simulink model "ROCR6II_URDF_file_915"  (R2020b)
settings: Solver=VariableStepAuto  StartTime=0.0  StopTime=10  FixedStep=0.01  RelTol=1e-3
values from neighbouring files (symbols this model uses):
  X = [x,y,z,Roll,Pitch,Yaw]    [T2RPY.m]
undefined symbols (not defined in the file or in its folder): A, Y, Z
libraries: fl_lib x115, sm_lib x74, nesl_utility x59, fl_ps_legacy_lib x48, ee_lib x12, simulink_extras x7, simulink x6
(part 1 of 5)
settings Model: Creator=Jeason  LastModifiedBy=GDXYY-006-F
settings DataIOCC: ReturnWorkspaceOutputs=off
settings DebuggingCC: ArithmeticOperatorsInVariantConditions=warning
settings SFSimCC: CustomCodeUndefinedFunction=UseInterfaceOnly

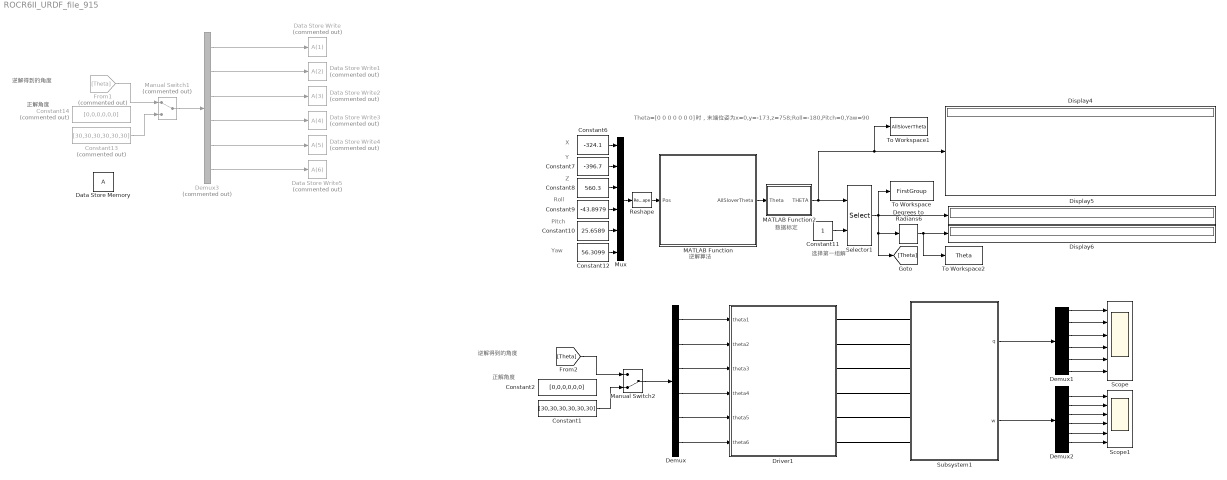
== system ROCR6II_URDF_file_915 ==
  note: 选择第一组解
  note: 数据标定
  note: Theta=[0 0 0 0 0 0 0]时，末端位姿为x=0,y=-173,z=758;Roll=-180,Pitch=0,Yaw=90
  note: 逆解算法
  note: 正解角度
  note: 逆解得到的角度
  note: Y
  note: Yaw
  note: Pitch
  note: Roll
  note: X
  note: Z
  note: 正解角度
  note: 逆解得到的角度
  Constant1 : Constant  Value=[30,30,30,30,30,30]
  Constant10 : Constant  Value=25.6589
  Constant11 : Constant
  Constant12 : Constant  Value=56.3099
  Constant13 : Constant  Commented=on  Value=[30,30,30,30,30,30]
  Constant14 : Constant  Commented=on  Value=[0,0,0,0,0,0]
  Constant2 : Constant  Value=[0,0,0,0,0,0]
  Constant6 : Constant  Value=-324.1
  Constant7 : Constant  Value=-396.7
  Constant8 : Constant  Value=560.3
  Constant9 : Constant  Value=-43.8979
  Data Store Write : DataStoreWrite  Commented=on  DataStoreElements=A(1)
  Data Store Write1 : DataStoreWrite  Commented=on  DataStoreElements=A(2)
  Data Store Write2 : DataStoreWrite  Commented=on  DataStoreElements=A(3)
  Data Store Write3 : DataStoreWrite  Commented=on  DataStoreElements=A(4)
  Data Store Write4 : DataStoreWrite  Commented=on  DataStoreElements=A(5)
  Data Store Write5 : DataStoreWrite  Commented=on  DataStoreElements=A(6)
  Data Store Memory : DataStoreMemory  ReadBeforeWriteMsg=warning  WriteAfterWriteMsg=warning  WriteAfterReadMsg=warning  InitialValue=[0 0 0 0 0 0]  ShowAdditionalParam=off
  Degrees to Radians6 : simulink_extras/Transformations/Degrees to Radians
  Demux : Demux  Outputs=6
  Demux1 : Demux  Outputs=6
  Demux2 : Demux  Outputs=6
  Demux3 : Demux  Commented=on  Outputs=6
  Display4 : Display
  Display5 : Display
  Display6 : Display
  Driver1 : Subsystem  mask{angle1=0, angle2=0, angle3=0, angle4=0, angle5=0, angle6=0}
      mask prompts: angle1 "InitTheta1(deg)"; angle2 "InitTheta2(deg)"; angle3 "InitTheta3(deg)"; angle4 "InitTheta4(deg)"; angle5 "InitTheta5(deg)"; angle6 "InitTheta6(deg)"
  From1 : From  Commented=on  GotoTag=Theta
  MATLAB Function : MATLAB Function  TreatAsAtomicUnit=on
  MATLAB Function2 : MATLAB Function  TreatAsAtomicUnit=on
  Manual Switch1 : ManualSwitch  Commented=on
  Manual Switch2 : ManualSwitch  CurrentSetting=0
  Mux : Mux  Inputs=6
  Reshape : Reshape  OutputDimensionality=Customize  OutputDimensions=[1,6]
  Scope : Scope  NumInputPorts=6
  Scope1 : Scope  NumInputPorts=6
  Selector1 : Selector  NumberOfDimensions=2  InputPortWidth=10  IndexOptions=Index vector (port),Starting index (dialog)  Indices=[1 3],1  OutputSizes=1,6
  Subsystem1 : Subsystem
  To Workspace : ToWorkspace  VariableName=FirstGroup  SampleTime=-1
      settings: MaxDataPoints=1
  To Workspace1 : ToWorkspace  VariableName=AllSloverTheta  SampleTime=-1
      settings: MaxDataPoints=1
  To Workspace2 : ToWorkspace  VariableName=Theta  SampleTime=-1
      settings: MaxDataPoints=1
  wires:
  Demux2/4 -> Scope1/4
  Demux1/4 -> Scope/4
  Demux2/6 -> Scope1/6
  Demux1/1 -> Scope/1
  Demux2/5 -> Scope1/5
  Demux2/1 -> Scope1/1
  Subsystem1/2(w) -> Demux2/1
  Demux2/3 -> Scope1/3
  Demux1/6 -> Scope/6
  Demux2/2 -> Scope1/2
  Demux1/2 -> Scope/2
  Subsystem1/1(q) -> Demux1/1
  Demux1/3 -> Scope/3
  Demux1/5 -> Scope/5
  Demux/1 -> Driver1/1(theta1)
  Demux/2 -> Driver1/2(theta2)
  Demux/3 -> Driver1/3(theta3)
  Demux/4 -> Driver1/4(theta4)
  Demux/5 -> Driver1/5(theta5)
  Demux/6 -> Driver1/6(theta6)
  Selector1/1 -> Display5/1, Degrees to Radians6/1, [Theta], To Workspace/1
  Degrees to Radians6/1 -> Display6/1, To Workspace2/1
  Reshape/1 -> MATLAB Function/1(Pos)
  Constant11/1 -> Selector1/2
  Mux/1 -> Reshape/1
  MATLAB Function/1(AllSloverTheta) -> MATLAB Function2/1(Theta)
  MATLAB Function2/1(THETA) -> Selector1/1, Display4/1, To Workspace1/1
  Constant13/1 -> Manual Switch1/2
  From1/1 -> Manual Switch1/1
  Demux3/4 -> Data Store Write3/1
  Demux3/6 -> Data Store Write5/1
  Demux3/1 -> Data Store Write/1
  Demux3/2 -> Data Store Write1/1
  Demux3/3 -> Data Store Write2/1
  Manual Switch1/1 -> Demux3/1
  Demux3/5 -> Data Store Write4/1
  Constant8/1 -> Mux/3
  Constant10/1 -> Mux/5
  Constant7/1 -> Mux/2
  Constant12/1 -> Mux/6
  Constant6/1 -> Mux/1
  Constant9/1 -> Mux/4
  Manual Switch2/1 -> Demux/1
  [Theta] -> Manual Switch2/1
  Constant1/1 -> Manual Switch2/2
  connections:
  Driver1/RConn1 -- Subsystem1/LConn1
  Driver1/RConn2 -- Subsystem1/LConn2
  Driver1/RConn3 -- Subsystem1/LConn3
  Driver1/RConn4 -- Subsystem1/LConn4
  Driver1/RConn5 -- Subsystem1/LConn5
  Driver1/RConn6 -- Subsystem1/LConn6

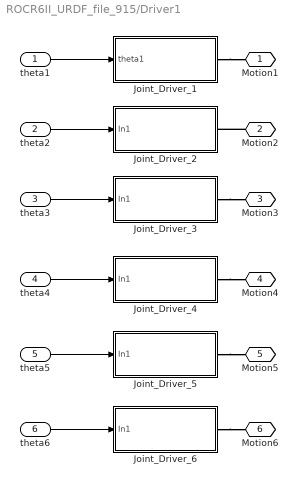
== system ROCR6II_URDF_file_915/Driver1 ==
  theta1 : Inport
  theta2 : Inport  Port=2
  theta3 : Inport  Port=3
  theta4 : Inport  Port=4
  theta5 : Inport  Port=5
  theta6 : Inport  Port=6
  Joint_Driver_1 : Subsystem
  Joint_Driver_2 : Subsystem
  Joint_Driver_3 : Subsystem
  Joint_Driver_4 : Subsystem
  Joint_Driver_5 : Subsystem
  Joint_Driver_6 : Subsystem
  Motion1 : PMIOPort  Side=Right
  Motion2 : PMIOPort  Port=2  Side=Right
  Motion3 : PMIOPort  Port=3  Side=Right
  Motion4 : PMIOPort  Port=4  Side=Right
  Motion5 : PMIOPort  Port=5  Side=Right
  Motion6 : PMIOPort  Port=6  Side=Right
  wires:
  theta2/1 -> Joint_Driver_2/1(In1)
  theta3/1 -> Joint_Driver_3/1(In1)
  theta4/1 -> Joint_Driver_4/1(In1)
  theta6/1 -> Joint_Driver_6/1(In1)
  theta5/1 -> Joint_Driver_5/1(In1)
  theta1/1 -> Joint_Driver_1/1(theta1)
  connections:
  Motion2/RConn1 -- Joint_Driver_2/RConn1
  Joint_Driver_6/RConn1 -- Motion6/RConn1
  Joint_Driver_1/RConn1 -- Motion1/RConn1
  Joint_Driver_3/RConn1 -- Motion3/RConn1
  Joint_Driver_5/RConn1 -- Motion5/RConn1
  Joint_Driver_4/RConn1 -- Motion4/RConn1

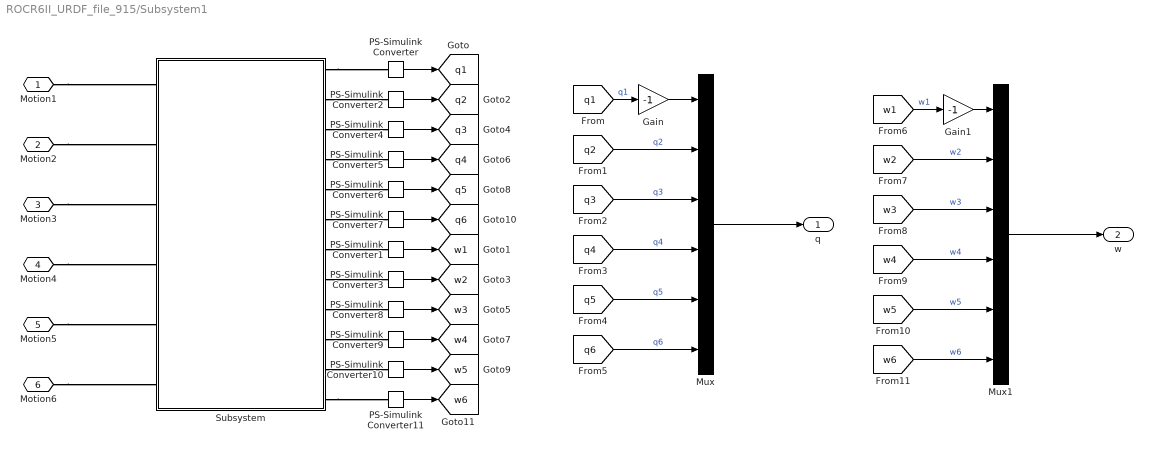
== system ROCR6II_URDF_file_915/Subsystem1 ==
  Gain : Gain  Gain=-1
  Gain1 : Gain  Gain=-1
  Mux : Mux  Inputs=6
  Mux1 : Mux  Inputs=6
  PS-Simulink Converter{,2,4..7} (6 alike) : nesl_utility/PS-Simulink Converter  PhysicalDomain=network_engine_domain  SubClassName=ps_output  LeftPortType=input  RightPortType=output  PseudoPeriodic=off  Frequencies=[]  Unit=deg  AffineConversion=off
  PS-Simulink Converter{1,3,8..11} (6 alike) : nesl_utility/PS-Simulink Converter  PhysicalDomain=network_engine_domain  SubClassName=ps_output  LeftPortType=input  RightPortType=output  PseudoPeriodic=off  Frequencies=[]  Unit=deg/s  AffineConversion=off
  Subsystem : Subsystem
  Motion1 : PMIOPort  Side=Left
  Motion2 : PMIOPort  Port=2  Side=Left
  Motion3 : PMIOPort  Port=3  Side=Left
  Motion4 : PMIOPort  Port=4  Side=Left
  Motion5 : PMIOPort  Port=5  Side=Left
  Motion6 : PMIOPort  Port=6  Side=Left
  q : Outport
  w : Outport  Port=2
  tag scope: q1=global, q2=global, q3=global, q4=global, q5=global, q6=global, w1=global, w2=global, w3=global, w4=global, w5=global, w6=global
  wires:
  [q2] -> Mux/2  "q2"
  PS-Simulink Converter11/1 -> [w6]
  PS-Simulink Converter1/1 -> [w1]
  Mux/1 -> q/1
  [w1] -> Gain1/1  "w1"
  PS-Simulink Converter6/1 -> [q5]
  [w4] -> Mux1/4  "w4"
  PS-Simulink Converter/1 -> [q1]
  [q6] -> Mux/6  "q6"
  PS-Simulink Converter7/1 -> [q6]
  [q3] -> Mux/3  "q3"
  [q4] -> Mux/4  "q4"
  PS-Simulink Converter10/1 -> [w5]
  PS-Simulink Converter4/1 -> [q3]
  PS-Simulink Converter2/1 -> [q2]
  [w2] -> Mux1/2  "w2"
  PS-Simulink Converter9/1 -> [w4]
  PS-Simulink Converter8/1 -> [w3]
  PS-Simulink Converter3/1 -> [w2]
  [w6] -> Mux1/6  "w6"
  Mux1/1 -> w/1
  [w5] -> Mux1/5  "w5"
  Gain1/1 -> Mux1/1
  PS-Simulink Converter5/1 -> [q4]
  Gain/1 -> Mux/1
  [w3] -> Mux1/3  "w3"
  [q1] -> Gain/1  "q1"
  [q5] -> Mux/5  "q5"
  connections:
  Subsystem/RConn12 -- PS-Simulink Converter11/LConn1
  Subsystem/RConn8 -- PS-Simulink Converter3/LConn1
  Subsystem/RConn4 -- PS-Simulink Converter5/LConn1
  Subsystem/RConn1 -- PS-Simulink Converter/LConn1
  Subsystem/RConn11 -- PS-Simulink Converter10/LConn1
  Subsystem/RConn2 -- PS-Simulink Converter2/LConn1
  Subsystem/RConn5 -- PS-Simulink Converter6/LConn1
  Subsystem/RConn3 -- PS-Simulink Converter4/LConn1
  Subsystem/RConn9 -- PS-Simulink Converter8/LConn1
  Subsystem/RConn7 -- PS-Simulink Converter1/LConn1
  Subsystem/RConn10 -- PS-Simulink Converter9/LConn1
  Subsystem/RConn6 -- PS-Simulink Converter7/LConn1
  Motion1/RConn1 -- Subsystem/LConn1
  Motion2/RConn1 -- Subsystem/LConn2
  Motion3/RConn1 -- Subsystem/LConn3
  Motion4/RConn1 -- Subsystem/LConn4
  Motion5/RConn1 -- Subsystem/LConn5
  Motion6/RConn1 -- Subsystem/LConn6

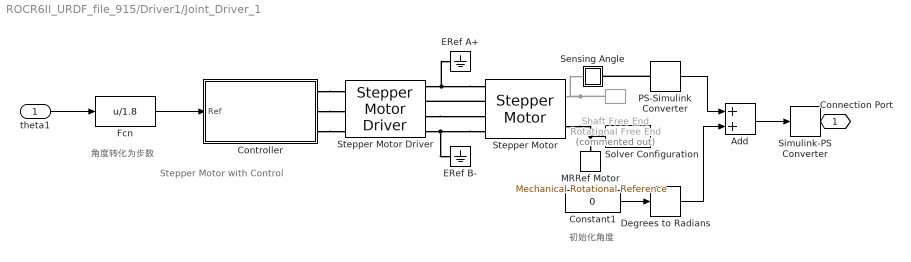
== system ROCR6II_URDF_file_915/Driver1/Joint_Driver_1 ==
  note: 初始化角度
  note: Stepper Motor with Control
  note: 角度转化为步数
  theta1 : Inport
  Add : Sum
  Constant1 : Constant  Value=0
  Controller : Subsystem  Variant=on  VariantControlMode=label  LabelModeActiveChoice=Position
      settings: AttributesFormatString=%<BlockChoice>
  Degrees to Radians : simulink_extras/Transformations/Degrees to Radians
  ERef A+ : fl_lib/Electrical/Electrical Elements/Electrical Reference
      settings: SourceProductName=Foundation Library
  ERef B- : fl_lib/Electrical/Electrical Elements/Electrical Reference
      settings: SourceProductName=Foundation Library
  Fcn : Fcn  Expr=u/1.8
  MRRef Motor : fl_lib/Mechanical/Rotational Elements/Mechanical Rotational Reference
      settings: SourceProductName=Foundation Library
  PS-Simulink Converter : nesl_utility/PS-Simulink Converter  PhysicalDomain=network_engine_domain  SubClassName=ps_output  LeftPortType=input  RightPortType=output  PseudoPeriodic=off  Frequencies=[]  Unit=1  AffineConversion=off
  Sensing Angle : Subsystem
      mask Display: disp('a')
  Shaft Free End : fl_lib/Mechanical/Rotational Elements/Rotational Free End  Commented=on  w_specify=off  w_priority=None  w=0 rad/s  w_nominal_specify=off  w_nominal_unit=rad/s  w_nominal_value=1
      settings: SourceProductName=Foundation Library
  Simulink-PS Converter : nesl_utility/Simulink-PS Converter  PhysicalDomain=network_engine_domain  SubClassName=ps_input  LeftPortType=input  RightPortType=output  PseudoPeriodic=off  Frequencies=[]  NoiseDistribution=none  NoiseParameters=[]  Unit=1  AffineConversion=off  FilteringAndDerivatives=filter  SimscapeFilterOrder=2  InputFilterTimeConstant=0.001  UdotUserProvided=0
  Solver Configuration : nesl_utility/Solver Configuration  PhysicalDomain=network_engine_domain  SubClassName=solver  LeftPortType=input  RightPortType=generic  Tones=[]  Harmonics=[]  SimulateNoise=off  Profile=off  UseLocalSampling=off  EnableSwitchedLinearOptims=on  FrequencyDomain=off  UseCCode=off  RelTol=0.001  AbsTol=1e-06  MinStep=1e-09  ToWorkspace=off  RevertToSquareIcSolve=off  NumHomotopyIterations=100  PhasorMode=off  PhasorModeNumHarmonics=1  DoDC=off  ResidualTolerance=1e-9  UseLocalSolver=off  LocalSolverChoice=NE_BACKWARD_EULER_ADVANCER  LocalSolverSampleTime=.001  DoFixedCost=off  MaxNonlinIter=3  MaxModeIter=2  ComputeImpulses=off  ImpulseIterations=2  LinearAlgebra=Sparse  EquationFormulation=NE_TIME_EF  DelaysMemoryBudget=1024  AutomaticFiltering=on  FilteringTimeConstant=0.001  PartitionStorageMethod=AS_NEEDED  PartitionMemoryBudget=1024  PartitionMethod=FAST
  Stepper Motor : ee_lib/Electromechanical/Reluctance & Stepper/Stepper Motor  step_or_av=1  w_vec=[ 0 1000 3e+3 ] rpm  T_vec=[ 2 2 1 ] N*m  assert_if_slipping=0  J_total=1e-4 kg*m^2  max_step_rate=10 Hz  Ra=0.55 Ohm  La=0.0015 H  Km=0.19 N*m/A  Td=0 N*m  Rm=Inf Ohm  Step=1.8 deg  J=4.5e-05 kg*m^2  B=1e-02 N*m/(rad/s)  speed0=0 rpm  theta0=0 deg  alpha=[.00393, .00393] 1/K  Tmeas=25 degC  T_vec2=[1.7, 1.7, .85] N*m  Tmeas2=125 degC  half_stepping=0  thermal_masses=[100, 100] J/K  initial_temperatures=[25, 25] degC  rotor_thermal_mass=50 J/K  rotor_initial_temperature=25 degC  Rm_percent_rotor=90
      settings: SourceProductBaseCode=PS  InternalSimscapePortConfiguration="{\"Bottom\":[],\"Left\":[{\"id\":\"pA\",\"label\":\"A+\",\"type\":\"foundation.electrical.electrical\"},{\"id\":\"nA\",\"label\":\"A-\",\"type\":\"foundation.electrical.electrical\"},{\"id\":\"pB\",\"label\":\"B+\",\"type\":\"foundation.electrical.electrical\"},{\"id\":\"nB\",\"label\":\"B-\",\"type\":\"foundation.electrical.electrical\"}],\"Right\":[{\"id\":\"R\",\"label\":\"R\",\"type\":\"foundation.mechanical.rotational.rotational\"},{\"id\":\"C\",\"label\":\"C\",\"type\":\"foundation.mechanical.rotational.rotational\"}],\"Top\":[]}"
  Stepper Motor Driver : ee_lib/Electromechanical/Reluctance & Stepper/Stepper Motor Driver  step_or_av=1  step_rate_per_volt=10 Hz/V  Venable=2.5 V  Vreverse=2.5 V  Vm=5 V  half_stepping=0
      settings: SourceProductBaseCode=PS  InternalSimscapePortConfiguration="{\"Bottom\":[],\"Left\":[{\"id\":\"ENA\",\"label\":\"ENA\",\"type\":\"foundation.electrical.electrical\"},{\"id\":\"REF\",\"label\":\"REF\",\"type\":\"foundation.electrical.electrical\"},{\"id\":\"REV\",\"label\":\"REV\",\"type\":\"foundation.electrical.electrical\"}],\"Right\":[{\"id\":\"pA\",\"label\":\"A+\",\"type\":\"foundation.electrical.electrical\"},{\"id\":\"nA\",\"label\":\"A-\",\"type\":\"foundation.electrical.electrical\"},{\"id\":\"pB\",\"label\":\"B+\",\"type\":\"foundation.electrical.electrical\"},{\"id\":\"nB\",\"label\":\"B-\",\"type\":\"foundation.electrical.electrical\"}],\"Top\":[]}"
  Connection Port : PMIOPort  Side=Right
  wires:
  Fcn/1 -> Controller/1(Ref)
  theta1/1 -> Fcn/1
  Constant1/1 -> Degrees to Radians/1
  PS-Simulink Converter/1 -> Add/1
  Add/1 -> Simulink-PS Converter/1
  Degrees to Radians/1 -> Add/2
  connections:
  PS-Simulink Converter/LConn1 -- Sensing Angle/RConn1
  Controller/RConn3 -- Stepper Motor Driver/LConn3
  Controller/RConn2 -- Stepper Motor Driver/LConn2
  Controller/RConn1 -- Stepper Motor Driver/LConn1
  Stepper Motor/LConn2 -- Stepper Motor Driver/RConn2
  Stepper Motor Driver/RConn3 -- Stepper Motor/LConn3
  Stepper Motor/LConn1 -- Stepper Motor Driver/RConn1 -- ERef A+/LConn1
  Solver Configuration/RConn1 -- Stepper Motor/RConn2 -- MRRef Motor/LConn1
  Shaft Free End/LConn1 -- Sensing Angle/LConn1 -- Stepper Motor/RConn1
  Stepper Motor/LConn4 -- Stepper Motor Driver/RConn4 -- ERef B-/LConn1
  Connection Port/RConn1 -- Simulink-PS Converter/RConn1

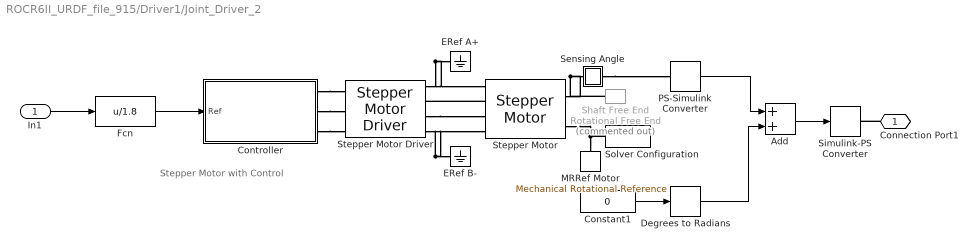
== system ROCR6II_URDF_file_915/Driver1/Joint_Driver_2 ==
  note: Stepper Motor with Control
  In1 : Inport
  Add : Sum
  Constant1 : Constant  Value=0
  Controller : Subsystem  Variant=on  VariantControlMode=label  LabelModeActiveChoice=Position
      settings: AttributesFormatString=%<BlockChoice>
  Degrees to Radians : simulink_extras/Transformations/Degrees to Radians
  ERef A+ : fl_lib/Electrical/Electrical Elements/Electrical Reference
      settings: SourceProductName=Foundation Library
  ERef B- : fl_lib/Electrical/Electrical Elements/Electrical Reference
      settings: SourceProductName=Foundation Library
  Fcn : Fcn  Expr=u/1.8
  MRRef Motor : fl_lib/Mechanical/Rotational Elements/Mechanical Rotational Reference
      settings: SourceProductName=Foundation Library
  PS-Simulink Converter : nesl_utility/PS-Simulink Converter  PhysicalDomain=network_engine_domain  SubClassName=ps_output  LeftPortType=input  RightPortType=output  PseudoPeriodic=off  Frequencies=[]  Unit=1  AffineConversion=off
  Sensing Angle : Subsystem
      mask Display: disp('a')
  Shaft Free End : fl_lib/Mechanical/Rotational Elements/Rotational Free End  Commented=on  w_specify=off  w_priority=None  w=0 rad/s  w_nominal_specify=off  w_nominal_unit=rad/s  w_nominal_value=1
      settings: SourceProductName=Foundation Library
  Simulink-PS Converter : nesl_utility/Simulink-PS Converter  PhysicalDomain=network_engine_domain  SubClassName=ps_input  LeftPortType=input  RightPortType=output  PseudoPeriodic=off  Frequencies=[]  NoiseDistribution=none  NoiseParameters=[]  Unit=1  AffineConversion=off  FilteringAndDerivatives=filter  SimscapeFilterOrder=2  InputFilterTimeConstant=0.001  UdotUserProvided=0
  Solver Configuration : nesl_utility/Solver Configuration  PhysicalDomain=network_engine_domain  SubClassName=solver  LeftPortType=input  RightPortType=generic  Tones=[]  Harmonics=[]  SimulateNoise=off  Profile=off  UseLocalSampling=off  EnableSwitchedLinearOptims=on  FrequencyDomain=off  UseCCode=off  RelTol=0.001  AbsTol=1e-06  MinStep=1e-09  ToWorkspace=off  RevertToSquareIcSolve=off  NumHomotopyIterations=100  PhasorMode=off  PhasorModeNumHarmonics=1  DoDC=off  ResidualTolerance=1e-9  UseLocalSolver=off  LocalSolverChoice=NE_BACKWARD_EULER_ADVANCER  LocalSolverSampleTime=.001  DoFixedCost=off  MaxNonlinIter=3  MaxModeIter=2  ComputeImpulses=off  ImpulseIterations=2  LinearAlgebra=Sparse  EquationFormulation=NE_TIME_EF  DelaysMemoryBudget=1024  AutomaticFiltering=on  FilteringTimeConstant=0.001  PartitionStorageMethod=AS_NEEDED  PartitionMemoryBudget=1024  PartitionMethod=FAST
  Stepper Motor : ee_lib/Electromechanical/Reluctance & Stepper/Stepper Motor  step_or_av=1  w_vec=[ 0 1000 3e+3 ] rpm  T_vec=[ 2 2 1 ] N*m  assert_if_slipping=0  J_total=1e-4 kg*m^2  max_step_rate=10 Hz  Ra=0.55 Ohm  La=0.0015 H  Km=0.19 N*m/A  Td=0 N*m  Rm=Inf Ohm  Step=1.8 deg  J=4.5e-05 kg*m^2  B=1e-02 N*m/(rad/s)  speed0=0 rpm  theta0=0 deg  alpha=[.00393, .00393] 1/K  Tmeas=25 degC  T_vec2=[1.7, 1.7, .85] N*m  Tmeas2=125 degC  half_stepping=0  thermal_masses=[100, 100] J/K  initial_temperatures=[25, 25] degC  rotor_thermal_mass=50 J/K  rotor_initial_temperature=25 degC  Rm_percent_rotor=90
      settings: SourceProductBaseCode=PS  InternalSimscapePortConfiguration="{\"Bottom\":[],\"Left\":[{\"id\":\"pA\",\"label\":\"A+\",\"type\":\"foundation.electrical.electrical\"},{\"id\":\"nA\",\"label\":\"A-\",\"type\":\"foundation.electrical.electrical\"},{\"id\":\"pB\",\"label\":\"B+\",\"type\":\"foundation.electrical.electrical\"},{\"id\":\"nB\",\"label\":\"B-\",\"type\":\"foundation.electrical.electrical\"}],\"Right\":[{\"id\":\"R\",\"label\":\"R\",\"type\":\"foundation.mechanical.rotational.rotational\"},{\"id\":\"C\",\"label\":\"C\",\"type\":\"foundation.mechanical.rotational.rotational\"}],\"Top\":[]}"
  Stepper Motor Driver : ee_lib/Electromechanical/Reluctance & Stepper/Stepper Motor Driver  step_or_av=1  step_rate_per_volt=10 Hz/V  Venable=2.5 V  Vreverse=2.5 V  Vm=5 V  half_stepping=0
      settings: SourceProductBaseCode=PS  InternalSimscapePortConfiguration="{\"Bottom\":[],\"Left\":[{\"id\":\"ENA\",\"label\":\"ENA\",\"type\":\"foundation.electrical.electrical\"},{\"id\":\"REF\",\"label\":\"REF\",\"type\":\"foundation.electrical.electrical\"},{\"id\":\"REV\",\"label\":\"REV\",\"type\":\"foundation.electrical.electrical\"}],\"Right\":[{\"id\":\"pA\",\"label\":\"A+\",\"type\":\"foundation.electrical.electrical\"},{\"id\":\"nA\",\"label\":\"A-\",\"type\":\"foundation.electrical.electrical\"},{\"id\":\"pB\",\"label\":\"B+\",\"type\":\"foundation.electrical.electrical\"},{\"id\":\"nB\",\"label\":\"B-\",\"type\":\"foundation.electrical.electrical\"}],\"Top\":[]}"
  Connection Port1 : PMIOPort  Side=Right
  wires:
  In1/1 -> Fcn/1
  Fcn/1 -> Controller/1(Ref)
  Add/1 -> Simulink-PS Converter/1
  Constant1/1 -> Degrees to Radians/1
  PS-Simulink Converter/1 -> Add/1
  Degrees to Radians/1 -> Add/2
  connections:
  ERef B-/LConn1 -- Stepper Motor Driver/RConn4 -- Stepper Motor/LConn4
  Sensing Angle/LConn1 -- Shaft Free End/LConn1 -- Stepper Motor/RConn1
  MRRef Motor/LConn1 -- Stepper Motor/RConn2 -- Solver Configuration/RConn1
  ERef A+/LConn1 -- Stepper Motor Driver/RConn1 -- Stepper Motor/LConn1
  Stepper Motor Driver/RConn3 -- Stepper Motor/LConn3
  Stepper Motor/LConn2 -- Stepper Motor Driver/RConn2
  Controller/RConn1 -- Stepper Motor Driver/LConn1
  Controller/RConn2 -- Stepper Motor Driver/LConn2
  Controller/RConn3 -- Stepper Motor Driver/LConn3
  Sensing Angle/RConn1 -- PS-Simulink Converter/LConn1
  Connection Port1/RConn1 -- Simulink-PS Converter/RConn1

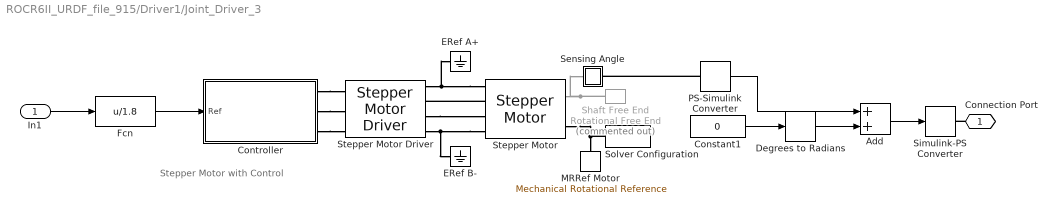
== system ROCR6II_URDF_file_915/Driver1/Joint_Driver_3 ==
  note: Stepper Motor with Control
  In1 : Inport
  Add : Sum
  Constant1 : Constant  Value=0
  Controller : Subsystem  Variant=on  VariantControlMode=label  LabelModeActiveChoice=Position
      settings: AttributesFormatString=%<BlockChoice>
  Degrees to Radians : simulink_extras/Transformations/Degrees to Radians
  ERef A+ : fl_lib/Electrical/Electrical Elements/Electrical Reference
      settings: SourceProductName=Foundation Library
  ERef B- : fl_lib/Electrical/Electrical Elements/Electrical Reference
      settings: SourceProductName=Foundation Library
  Fcn : Fcn  Expr=u/1.8
  MRRef Motor : fl_lib/Mechanical/Rotational Elements/Mechanical Rotational Reference
      settings: SourceProductName=Foundation Library
  PS-Simulink Converter : nesl_utility/PS-Simulink Converter  PhysicalDomain=network_engine_domain  SubClassName=ps_output  LeftPortType=input  RightPortType=output  PseudoPeriodic=off  Frequencies=[]  Unit=1  AffineConversion=off
  Sensing Angle : Subsystem
      mask Display: disp('a')
  Shaft Free End : fl_lib/Mechanical/Rotational Elements/Rotational Free End  Commented=on  w_specify=off  w_priority=None  w=0 rad/s  w_nominal_specify=off  w_nominal_unit=rad/s  w_nominal_value=1
      settings: SourceProductName=Foundation Library
  Simulink-PS Converter : nesl_utility/Simulink-PS Converter  PhysicalDomain=network_engine_domain  SubClassName=ps_input  LeftPortType=input  RightPortType=output  PseudoPeriodic=off  Frequencies=[]  NoiseDistribution=none  NoiseParameters=[]  Unit=1  AffineConversion=off  FilteringAndDerivatives=filter  SimscapeFilterOrder=2  InputFilterTimeConstant=0.001  UdotUserProvided=0
  Solver Configuration : nesl_utility/Solver Configuration  PhysicalDomain=network_engine_domain  SubClassName=solver  LeftPortType=input  RightPortType=generic  Tones=[]  Harmonics=[]  SimulateNoise=off  Profile=off  UseLocalSampling=off  EnableSwitchedLinearOptims=on  FrequencyDomain=off  UseCCode=off  RelTol=0.001  AbsTol=1e-06  MinStep=1e-09  ToWorkspace=off  RevertToSquareIcSolve=off  NumHomotopyIterations=100  PhasorMode=off  PhasorModeNumHarmonics=1  DoDC=off  ResidualTolerance=1e-9  UseLocalSolver=off  LocalSolverChoice=NE_BACKWARD_EULER_ADVANCER  LocalSolverSampleTime=.001  DoFixedCost=off  MaxNonlinIter=3  MaxModeIter=2  ComputeImpulses=off  ImpulseIterations=2  LinearAlgebra=Sparse  EquationFormulation=NE_TIME_EF  DelaysMemoryBudget=1024  AutomaticFiltering=on  FilteringTimeConstant=0.001  PartitionStorageMethod=AS_NEEDED  PartitionMemoryBudget=1024  PartitionMethod=FAST
  Stepper Motor : ee_lib/Electromechanical/Reluctance & Stepper/Stepper Motor  step_or_av=1  w_vec=[ 0 1000 3e+3 ] rpm  T_vec=[ 2 2 1 ] N*m  assert_if_slipping=0  J_total=1e-4 kg*m^2  max_step_rate=10 Hz  Ra=0.55 Ohm  La=0.0015 H  Km=0.19 N*m/A  Td=0 N*m  Rm=Inf Ohm  Step=1.8 deg  J=4.5e-05 kg*m^2  B=1e-02 N*m/(rad/s)  speed0=0 rpm  theta0=0 deg  alpha=[.00393, .00393] 1/K  Tmeas=25 degC  T_vec2=[1.7, 1.7, .85] N*m  Tmeas2=125 degC  half_stepping=0  thermal_masses=[100, 100] J/K  initial_temperatures=[25, 25] degC  rotor_thermal_mass=50 J/K  rotor_initial_temperature=25 degC  Rm_percent_rotor=90
      settings: SourceProductBaseCode=PS  InternalSimscapePortConfiguration="{\"Bottom\":[],\"Left\":[{\"id\":\"pA\",\"label\":\"A+\",\"type\":\"foundation.electrical.electrical\"},{\"id\":\"nA\",\"label\":\"A-\",\"type\":\"foundation.electrical.electrical\"},{\"id\":\"pB\",\"label\":\"B+\",\"type\":\"foundation.electrical.electrical\"},{\"id\":\"nB\",\"label\":\"B-\",\"type\":\"foundation.electrical.electrical\"}],\"Right\":[{\"id\":\"R\",\"label\":\"R\",\"type\":\"foundation.mechanical.rotational.rotational\"},{\"id\":\"C\",\"label\":\"C\",\"type\":\"foundation.mechanical.rotational.rotational\"}],\"Top\":[]}"
  Stepper Motor Driver : ee_lib/Electromechanical/Reluctance & Stepper/Stepper Motor Driver  step_or_av=1  step_rate_per_volt=10 Hz/V  Venable=2.5 V  Vreverse=2.5 V  Vm=5 V  half_stepping=0
      settings: SourceProductBaseCode=PS  InternalSimscapePortConfiguration="{\"Bottom\":[],\"Left\":[{\"id\":\"ENA\",\"label\":\"ENA\",\"type\":\"foundation.electrical.electrical\"},{\"id\":\"REF\",\"label\":\"REF\",\"type\":\"foundation.electrical.electrical\"},{\"id\":\"REV\",\"label\":\"REV\",\"type\":\"foundation.electrical.electrical\"}],\"Right\":[{\"id\":\"pA\",\"label\":\"A+\",\"type\":\"foundation.electrical.electrical\"},{\"id\":\"nA\",\"label\":\"A-\",\"type\":\"foundation.electrical.electrical\"},{\"id\":\"pB\",\"label\":\"B+\",\"type\":\"foundation.electrical.electrical\"},{\"id\":\"nB\",\"label\":\"B-\",\"type\":\"foundation.electrical.electrical\"}],\"Top\":[]}"
  Connection Port : PMIOPort  Side=Right
  wires:
  Fcn/1 -> Controller/1(Ref)
  In1/1 -> Fcn/1
  Add/1 -> Simulink-PS Converter/1
  Constant1/1 -> Degrees to Radians/1
  PS-Simulink Converter/1 -> Add/1
  Degrees to Radians/1 -> Add/2
  connections:
  PS-Simulink Converter/LConn1 -- Sensing Angle/RConn1
  Controller/RConn3 -- Stepper Motor Driver/LConn3
  Controller/RConn2 -- Stepper Motor Driver/LConn2
  Controller/RConn1 -- Stepper Motor Driver/LConn1
  Stepper Motor/LConn2 -- Stepper Motor Driver/RConn2
  Stepper Motor Driver/RConn3 -- Stepper Motor/LConn3
  Stepper Motor/LConn1 -- Stepper Motor Driver/RConn1 -- ERef A+/LConn1
  Solver Configuration/RConn1 -- Stepper Motor/RConn2 -- MRRef Motor/LConn1
  Shaft Free End/LConn1 -- Sensing Angle/LConn1 -- Stepper Motor/RConn1
  Stepper Motor/LConn4 -- Stepper Motor Driver/RConn4 -- ERef B-/LConn1
  Connection Port/RConn1 -- Simulink-PS Converter/RConn1

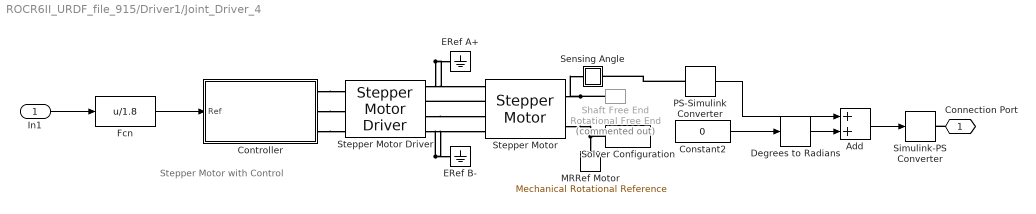
== system ROCR6II_URDF_file_915/Driver1/Joint_Driver_4 ==
  note: Stepper Motor with Control
  In1 : Inport
  Add : Sum
  Constant2 : Constant  Value=0
  Controller : Subsystem  Variant=on  VariantControlMode=label  LabelModeActiveChoice=Position
      settings: AttributesFormatString=%<BlockChoice>
  Degrees to Radians : simulink_extras/Transformations/Degrees to Radians
  ERef A+ : fl_lib/Electrical/Electrical Elements/Electrical Reference
      settings: SourceProductName=Foundation Library
  ERef B- : fl_lib/Electrical/Electrical Elements/Electrical Reference
      settings: SourceProductName=Foundation Library
  Fcn : Fcn  Expr=u/1.8
  MRRef Motor : fl_lib/Mechanical/Rotational Elements/Mechanical Rotational Reference
      settings: SourceProductName=Foundation Library
  PS-Simulink Converter : nesl_utility/PS-Simulink Converter  PhysicalDomain=network_engine_domain  SubClassName=ps_output  LeftPortType=input  RightPortType=output  PseudoPeriodic=off  Frequencies=[]  Unit=1  AffineConversion=off
  Sensing Angle : Subsystem
      mask Display: disp('a')
  Shaft Free End : fl_lib/Mechanical/Rotational Elements/Rotational Free End  Commented=on  w_specify=off  w_priority=None  w=0 rad/s  w_nominal_specify=off  w_nominal_unit=rad/s  w_nominal_value=1
      settings: SourceProductName=Foundation Library
  Simulink-PS Converter : nesl_utility/Simulink-PS Converter  PhysicalDomain=network_engine_domain  SubClassName=ps_input  LeftPortType=input  RightPortType=output  PseudoPeriodic=off  Frequencies=[]  NoiseDistribution=none  NoiseParameters=[]  Unit=1  AffineConversion=off  FilteringAndDerivatives=filter  SimscapeFilterOrder=2  InputFilterTimeConstant=0.001  UdotUserProvided=0
  Solver Configuration : nesl_utility/Solver Configuration  PhysicalDomain=network_engine_domain  SubClassName=solver  LeftPortType=input  RightPortType=generic  Tones=[]  Harmonics=[]  SimulateNoise=off  Profile=off  UseLocalSampling=off  EnableSwitchedLinearOptims=on  FrequencyDomain=off  UseCCode=off  RelTol=0.001  AbsTol=1e-06  MinStep=1e-09  ToWorkspace=off  RevertToSquareIcSolve=off  NumHomotopyIterations=100  PhasorMode=off  PhasorModeNumHarmonics=1  DoDC=off  ResidualTolerance=1e-9  UseLocalSolver=off  LocalSolverChoice=NE_BACKWARD_EULER_ADVANCER  LocalSolverSampleTime=.001  DoFixedCost=off  MaxNonlinIter=3  MaxModeIter=2  ComputeImpulses=off  ImpulseIterations=2  LinearAlgebra=Sparse  EquationFormulation=NE_TIME_EF  DelaysMemoryBudget=1024  AutomaticFiltering=on  FilteringTimeConstant=0.001  PartitionStorageMethod=AS_NEEDED  PartitionMemoryBudget=1024  PartitionMethod=FAST
  Stepper Motor : ee_lib/Electromechanical/Reluctance & Stepper/Stepper Motor  step_or_av=1  w_vec=[ 0 1000 3e+3 ] rpm  T_vec=[ 2 2 1 ] N*m  assert_if_slipping=0  J_total=1e-4 kg*m^2  max_step_rate=10 Hz  Ra=0.55 Ohm  La=0.0015 H  Km=0.19 N*m/A  Td=0 N*m  Rm=Inf Ohm  Step=1.8 deg  J=4.5e-05 kg*m^2  B=1e-02 N*m/(rad/s)  speed0=0 rpm  theta0=0 deg  alpha=[.00393, .00393] 1/K  Tmeas=25 degC  T_vec2=[1.7, 1.7, .85] N*m  Tmeas2=125 degC  half_stepping=0  thermal_masses=[100, 100] J/K  initial_temperatures=[25, 25] degC  rotor_thermal_mass=50 J/K  rotor_initial_temperature=25 degC  Rm_percent_rotor=90
      settings: SourceProductBaseCode=PS  InternalSimscapePortConfiguration="{\"Bottom\":[],\"Left\":[{\"id\":\"pA\",\"label\":\"A+\",\"type\":\"foundation.electrical.electrical\"},{\"id\":\"nA\",\"label\":\"A-\",\"type\":\"foundation.electrical.electrical\"},{\"id\":\"pB\",\"label\":\"B+\",\"type\":\"foundation.electrical.electrical\"},{\"id\":\"nB\",\"label\":\"B-\",\"type\":\"foundation.electrical.electrical\"}],\"Right\":[{\"id\":\"R\",\"label\":\"R\",\"type\":\"foundation.mechanical.rotational.rotational\"},{\"id\":\"C\",\"label\":\"C\",\"type\":\"foundation.mechanical.rotational.rotational\"}],\"Top\":[]}"
  Stepper Motor Driver : ee_lib/Electromechanical/Reluctance & Stepper/Stepper Motor Driver  step_or_av=1  step_rate_per_volt=10 Hz/V  Venable=2.5 V  Vreverse=2.5 V  Vm=5 V  half_stepping=0
      settings: SourceProductBaseCode=PS  InternalSimscapePortConfiguration="{\"Bottom\":[],\"Left\":[{\"id\":\"ENA\",\"label\":\"ENA\",\"type\":\"foundation.electrical.electrical\"},{\"id\":\"REF\",\"label\":\"REF\",\"type\":\"foundation.electrical.electrical\"},{\"id\":\"REV\",\"label\":\"REV\",\"type\":\"foundation.electrical.electrical\"}],\"Right\":[{\"id\":\"pA\",\"label\":\"A+\",\"type\":\"foundation.electrical.electrical\"},{\"id\":\"nA\",\"label\":\"A-\",\"type\":\"foundation.electrical.electrical\"},{\"id\":\"pB\",\"label\":\"B+\",\"type\":\"foundation.electrical.electrical\"},{\"id\":\"nB\",\"label\":\"B-\",\"type\":\"foundation.electrical.electrical\"}],\"Top\":[]}"
  Connection Port : PMIOPort  Side=Right
  wires:
  In1/1 -> Fcn/1
  Fcn/1 -> Controller/1(Ref)
  Add/1 -> Simulink-PS Converter/1
  Constant2/1 -> Degrees to Radians/1
  PS-Simulink Converter/1 -> Add/1
  Degrees to Radians/1 -> Add/2
  connections:
  ERef B-/LConn1 -- Stepper Motor Driver/RConn4 -- Stepper Motor/LConn4
  Stepper Motor/RConn1 -- Sensing Angle/LConn1 -- Shaft Free End/LConn1
  MRRef Motor/LConn1 -- Stepper Motor/RConn2 -- Solver Configuration/RConn1
  ERef A+/LConn1 -- Stepper Motor Driver/RConn1 -- Stepper Motor/LConn1
  Stepper Motor Driver/RConn3 -- Stepper Motor/LConn3
  Stepper Motor/LConn2 -- Stepper Motor Driver/RConn2
  Controller/RConn1 -- Stepper Motor Driver/LConn1
  Controller/RConn2 -- Stepper Motor Driver/LConn2
  Controller/RConn3 -- Stepper Motor Driver/LConn3
  PS-Simulink Converter/LConn1 -- Sensing Angle/RConn1
  Connection Port/RConn1 -- Simulink-PS Converter/RConn1

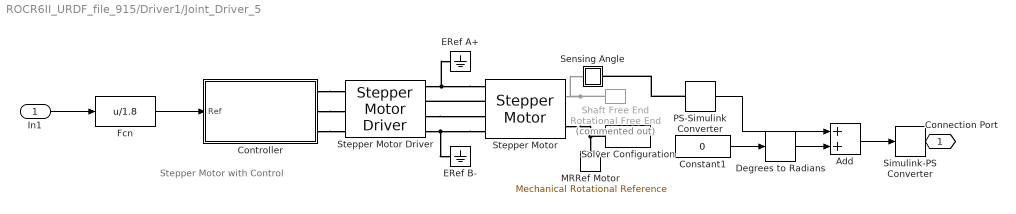
== system ROCR6II_URDF_file_915/Driver1/Joint_Driver_5 ==
  note: Stepper Motor with Control
  In1 : Inport
  Add : Sum
  Constant1 : Constant  Value=0
  Controller : Subsystem  Variant=on  VariantControlMode=label  LabelModeActiveChoice=Position
      settings: AttributesFormatString=%<BlockChoice>
  Degrees to Radians : simulink_extras/Transformations/Degrees to Radians
  ERef A+ : fl_lib/Electrical/Electrical Elements/Electrical Reference
      settings: SourceProductName=Foundation Library
  ERef B- : fl_lib/Electrical/Electrical Elements/Electrical Reference
      settings: SourceProductName=Foundation Library
  Fcn : Fcn  Expr=u/1.8
  MRRef Motor : fl_lib/Mechanical/Rotational Elements/Mechanical Rotational Reference
      settings: SourceProductName=Foundation Library
  PS-Simulink Converter : nesl_utility/PS-Simulink Converter  PhysicalDomain=network_engine_domain  SubClassName=ps_output  LeftPortType=input  RightPortType=output  PseudoPeriodic=off  Frequencies=[]  Unit=1  AffineConversion=off
  Sensing Angle : Subsystem
      mask Display: disp('a')
  Shaft Free End : fl_lib/Mechanical/Rotational Elements/Rotational Free End  Commented=on  w_specify=off  w_priority=None  w=0 rad/s  w_nominal_specify=off  w_nominal_unit=rad/s  w_nominal_value=1
      settings: SourceProductName=Foundation Library
  Simulink-PS Converter : nesl_utility/Simulink-PS Converter  PhysicalDomain=network_engine_domain  SubClassName=ps_input  LeftPortType=input  RightPortType=output  PseudoPeriodic=off  Frequencies=[]  NoiseDistribution=none  NoiseParameters=[]  Unit=1  AffineConversion=off  FilteringAndDerivatives=filter  SimscapeFilterOrder=2  InputFilterTimeConstant=0.001  UdotUserProvided=0
  Solver Configuration : nesl_utility/Solver Configuration  PhysicalDomain=network_engine_domain  SubClassName=solver  LeftPortType=input  RightPortType=generic  Tones=[]  Harmonics=[]  SimulateNoise=off  Profile=off  UseLocalSampling=off  EnableSwitchedLinearOptims=on  FrequencyDomain=off  UseCCode=off  RelTol=0.001  AbsTol=1e-06  MinStep=1e-09  ToWorkspace=off  RevertToSquareIcSolve=off  NumHomotopyIterations=100  PhasorMode=off  PhasorModeNumHarmonics=1  DoDC=off  ResidualTolerance=1e-9  UseLocalSolver=off  LocalSolverChoice=NE_BACKWARD_EULER_ADVANCER  LocalSolverSampleTime=.001  DoFixedCost=off  MaxNonlinIter=3  MaxModeIter=2  ComputeImpulses=off  ImpulseIterations=2  LinearAlgebra=Sparse  EquationFormulation=NE_TIME_EF  DelaysMemoryBudget=1024  AutomaticFiltering=on  FilteringTimeConstant=0.001  PartitionStorageMethod=AS_NEEDED  PartitionMemoryBudget=1024  PartitionMethod=FAST
  Stepper Motor : ee_lib/Electromechanical/Reluctance & Stepper/Stepper Motor  step_or_av=1  w_vec=[ 0 1000 3e+3 ] rpm  T_vec=[ 2 2 1 ] N*m  assert_if_slipping=0  J_total=1e-4 kg*m^2  max_step_rate=10 Hz  Ra=0.55 Ohm  La=0.0015 H  Km=0.19 N*m/A  Td=0 N*m  Rm=Inf Ohm  Step=1.8 deg  J=4.5e-05 kg*m^2  B=1e-02 N*m/(rad/s)  speed0=0 rpm  theta0=0 deg  alpha=[.00393, .00393] 1/K  Tmeas=25 degC  T_vec2=[1.7, 1.7, .85] N*m  Tmeas2=125 degC  half_stepping=0  thermal_masses=[100, 100] J/K  initial_temperatures=[25, 25] degC  rotor_thermal_mass=50 J/K  rotor_initial_temperature=25 degC  Rm_percent_rotor=90
      settings: SourceProductBaseCode=PS  InternalSimscapePortConfiguration="{\"Bottom\":[],\"Left\":[{\"id\":\"pA\",\"label\":\"A+\",\"type\":\"foundation.electrical.electrical\"},{\"id\":\"nA\",\"label\":\"A-\",\"type\":\"foundation.electrical.electrical\"},{\"id\":\"pB\",\"label\":\"B+\",\"type\":\"foundation.electrical.electrical\"},{\"id\":\"nB\",\"label\":\"B-\",\"type\":\"foundation.electrical.electrical\"}],\"Right\":[{\"id\":\"R\",\"label\":\"R\",\"type\":\"foundation.mechanical.rotational.rotational\"},{\"id\":\"C\",\"label\":\"C\",\"type\":\"foundation.mechanical.rotational.rotational\"}],\"Top\":[]}"
  Stepper Motor Driver : ee_lib/Electromechanical/Reluctance & Stepper/Stepper Motor Driver  step_or_av=1  step_rate_per_volt=10 Hz/V  Venable=2.5 V  Vreverse=2.5 V  Vm=5 V  half_stepping=0
      settings: SourceProductBaseCode=PS  InternalSimscapePortConfiguration="{\"Bottom\":[],\"Left\":[{\"id\":\"ENA\",\"label\":\"ENA\",\"type\":\"foundation.electrical.electrical\"},{\"id\":\"REF\",\"label\":\"REF\",\"type\":\"foundation.electrical.electrical\"},{\"id\":\"REV\",\"label\":\"REV\",\"type\":\"foundation.electrical.electrical\"}],\"Right\":[{\"id\":\"pA\",\"label\":\"A+\",\"type\":\"foundation.electrical.electrical\"},{\"id\":\"nA\",\"label\":\"A-\",\"type\":\"foundation.electrical.electrical\"},{\"id\":\"pB\",\"label\":\"B+\",\"type\":\"foundation.electrical.electrical\"},{\"id\":\"nB\",\"label\":\"B-\",\"type\":\"foundation.electrical.electrical\"}],\"Top\":[]}"
  Connection Port : PMIOPort  Side=Right
  wires:
  Fcn/1 -> Controller/1(Ref)
  In1/1 -> Fcn/1
  Add/1 -> Simulink-PS Converter/1
  Constant1/1 -> Degrees to Radians/1
  PS-Simulink Converter/1 -> Add/1
  Degrees to Radians/1 -> Add/2
  connections:
  PS-Simulink Converter/LConn1 -- Sensing Angle/RConn1
  Controller/RConn3 -- Stepper Motor Driver/LConn3
  Controller/RConn2 -- Stepper Motor Driver/LConn2
  Controller/RConn1 -- Stepper Motor Driver/LConn1
  Stepper Motor/LConn2 -- Stepper Motor Driver/RConn2
  Stepper Motor Driver/RConn3 -- Stepper Motor/LConn3
  Stepper Motor/LConn1 -- Stepper Motor Driver/RConn1 -- ERef A+/LConn1
  Solver Configuration/RConn1 -- Stepper Motor/RConn2 -- MRRef Motor/LConn1
  Shaft Free End/LConn1 -- Sensing Angle/LConn1 -- Stepper Motor/RConn1
  Stepper Motor/LConn4 -- Stepper Motor Driver/RConn4 -- ERef B-/LConn1
  Connection Port/RConn1 -- Simulink-PS Converter/RConn1

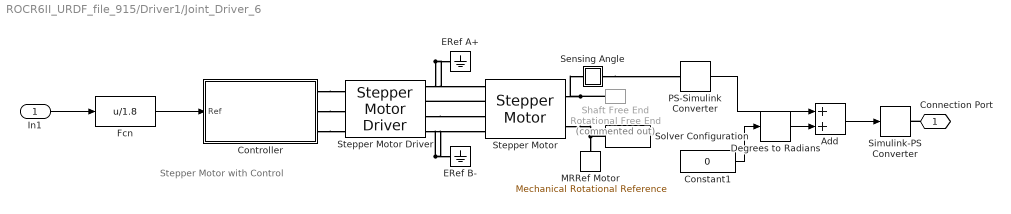
== system ROCR6II_URDF_file_915/Driver1/Joint_Driver_6 ==
  note: Stepper Motor with Control
  In1 : Inport
  Add : Sum
  Constant1 : Constant  Value=0
  Controller : Subsystem  Variant=on  VariantControlMode=label  LabelModeActiveChoice=Position
      settings: AttributesFormatString=%<BlockChoice>
  Degrees to Radians : simulink_extras/Transformations/Degrees to Radians
  ERef A+ : fl_lib/Electrical/Electrical Elements/Electrical Reference
      settings: SourceProductName=Foundation Library
  ERef B- : fl_lib/Electrical/Electrical Elements/Electrical Reference
      settings: SourceProductName=Foundation Library
  Fcn : Fcn  Expr=u/1.8
  MRRef Motor : fl_lib/Mechanical/Rotational Elements/Mechanical Rotational Reference
      settings: SourceProductName=Foundation Library
  PS-Simulink Converter : nesl_utility/PS-Simulink Converter  PhysicalDomain=network_engine_domain  SubClassName=ps_output  LeftPortType=input  RightPortType=output  PseudoPeriodic=off  Frequencies=[]  Unit=1  AffineConversion=off
  Sensing Angle : Subsystem
      mask Display: disp('a')
  Shaft Free End : fl_lib/Mechanical/Rotational Elements/Rotational Free End  Commented=on  w_specify=off  w_priority=None  w=0 rad/s  w_nominal_specify=off  w_nominal_unit=rad/s  w_nominal_value=1
      settings: SourceProductName=Foundation Library
  Simulink-PS Converter : nesl_utility/Simulink-PS Converter  PhysicalDomain=network_engine_domain  SubClassName=ps_input  LeftPortType=input  RightPortType=output  PseudoPeriodic=off  Frequencies=[]  NoiseDistribution=none  NoiseParameters=[]  Unit=1  AffineConversion=off  FilteringAndDerivatives=filter  SimscapeFilterOrder=2  InputFilterTimeConstant=0.001  UdotUserProvided=0
  Solver Configuration : nesl_utility/Solver Configuration  PhysicalDomain=network_engine_domain  SubClassName=solver  LeftPortType=input  RightPortType=generic  Tones=[]  Harmonics=[]  SimulateNoise=off  Profile=off  UseLocalSampling=off  EnableSwitchedLinearOptims=on  FrequencyDomain=off  UseCCode=off  RelTol=0.001  AbsTol=1e-06  MinStep=1e-09  ToWorkspace=off  RevertToSquareIcSolve=off  NumHomotopyIterations=100  PhasorMode=off  PhasorModeNumHarmonics=1  DoDC=off  ResidualTolerance=1e-9  UseLocalSolver=off  LocalSolverChoice=NE_BACKWARD_EULER_ADVANCER  LocalSolverSampleTime=.001  DoFixedCost=off  MaxNonlinIter=3  MaxModeIter=2  ComputeImpulses=off  ImpulseIterations=2  LinearAlgebra=Sparse  EquationFormulation=NE_TIME_EF  DelaysMemoryBudget=1024  AutomaticFiltering=on  FilteringTimeConstant=0.001  PartitionStorageMethod=AS_NEEDED  PartitionMemoryBudget=1024  PartitionMethod=FAST
  Stepper Motor : ee_lib/Electromechanical/Reluctance & Stepper/Stepper Motor  step_or_av=1  w_vec=[ 0 1000 3e+3 ] rpm  T_vec=[ 2 2 1 ] N*m  assert_if_slipping=0  J_total=1e-4 kg*m^2  max_step_rate=10 Hz  Ra=0.55 Ohm  La=0.0015 H  Km=0.19 N*m/A  Td=0 N*m  Rm=Inf Ohm  Step=1.8 deg  J=4.5e-05 kg*m^2  B=1e-02 N*m/(rad/s)  speed0=0 rpm  theta0=0 deg  alpha=[.00393, .00393] 1/K  Tmeas=25 degC  T_vec2=[1.7, 1.7, .85] N*m  Tmeas2=125 degC  half_stepping=0  thermal_masses=[100, 100] J/K  initial_temperatures=[25, 25] degC  rotor_thermal_mass=50 J/K  rotor_initial_temperature=25 degC  Rm_percent_rotor=90
      settings: SourceProductBaseCode=PS  InternalSimscapePortConfiguration="{\"Bottom\":[],\"Left\":[{\"id\":\"pA\",\"label\":\"A+\",\"type\":\"foundation.electrical.electrical\"},{\"id\":\"nA\",\"label\":\"A-\",\"type\":\"foundation.electrical.electrical\"},{\"id\":\"pB\",\"label\":\"B+\",\"type\":\"foundation.electrical.electrical\"},{\"id\":\"nB\",\"label\":\"B-\",\"type\":\"foundation.electrical.electrical\"}],\"Right\":[{\"id\":\"R\",\"label\":\"R\",\"type\":\"foundation.mechanical.rotational.rotational\"},{\"id\":\"C\",\"label\":\"C\",\"type\":\"foundation.mechanical.rotational.rotational\"}],\"Top\":[]}"
  Stepper Motor Driver : ee_lib/Electromechanical/Reluctance & Stepper/Stepper Motor Driver  step_or_av=1  step_rate_per_volt=10 Hz/V  Venable=2.5 V  Vreverse=2.5 V  Vm=5 V  half_stepping=0
      settings: SourceProductBaseCode=PS  InternalSimscapePortConfiguration="{\"Bottom\":[],\"Left\":[{\"id\":\"ENA\",\"label\":\"ENA\",\"type\":\"foundation.electrical.electrical\"},{\"id\":\"REF\",\"label\":\"REF\",\"type\":\"foundation.electrical.electrical\"},{\"id\":\"REV\",\"label\":\"REV\",\"type\":\"foundation.electrical.electrical\"}],\"Right\":[{\"id\":\"pA\",\"label\":\"A+\",\"type\":\"foundation.electrical.electrical\"},{\"id\":\"nA\",\"label\":\"A-\",\"type\":\"foundation.electrical.electrical\"},{\"id\":\"pB\",\"label\":\"B+\",\"type\":\"foundation.electrical.electrical\"},{\"id\":\"nB\",\"label\":\"B-\",\"type\":\"foundation.electrical.electrical\"}],\"Top\":[]}"
  Connection Port : PMIOPort  Side=Right
  wires:
  In1/1 -> Fcn/1
  Fcn/1 -> Controller/1(Ref)
  Add/1 -> Simulink-PS Converter/1
  Constant1/1 -> Degrees to Radians/1
  PS-Simulink Converter/1 -> Add/1
  Degrees to Radians/1 -> Add/2
  connections:
  ERef B-/LConn1 -- Stepper Motor Driver/RConn4 -- Stepper Motor/LConn4
  Stepper Motor/RConn1 -- Sensing Angle/LConn1 -- Shaft Free End/LConn1
  MRRef Motor/LConn1 -- Stepper Motor/RConn2 -- Solver Configuration/RConn1
  ERef A+/LConn1 -- Stepper Motor Driver/RConn1 -- Stepper Motor/LConn1
  Stepper Motor Driver/RConn3 -- Stepper Motor/LConn3
  Stepper Motor/LConn2 -- Stepper Motor Driver/RConn2
  Controller/RConn1 -- Stepper Motor Driver/LConn1
  Controller/RConn2 -- Stepper Motor Driver/LConn2
  Controller/RConn3 -- Stepper Motor Driver/LConn3
  Sensing Angle/RConn1 -- PS-Simulink Converter/LConn1
  Connection Port/RConn1 -- Simulink-PS Converter/RConn1
